simulink model "lane_departure"  (R2017a)
settings: Solver=FixedStepDiscrete  StartTime=0.0  StopTime=inf  FixedStep=1/50  RelTol=1e-3  EnableMultiTasking=on
libraries: visionsinks x1, dspvision x1, embdlinuxlib x1
settings Model: Creator=ChiChaChai  LastModifiedBy=ChiChaChai
settings SolverCC: PositivePriorityOrder=on  AutoInsertRateTranBlk=on
settings OptimizationCC: UseFloatMulNetSlope=on  PassReuseOutputArgsAs=Individual arguments  ZeroExternalMemoryAtStartup=off  ZeroInternalMemoryAtStartup=off  NoFixptDivByZeroProtection=on  EfficientFloat2IntCast=on  LifeSpan=1  MaxStackSize=64
settings DebuggingCC: ParameterTunabilityLossMsg=error
settings HardwareCC: ProdBitPerPointer=32  ProdBitPerSizeT=32  ProdBitPerPtrDiffT=32  ProdLargestAtomicInteger=Long  ProdLargestAtomicFloat=Double  ProdWordSize=32  ProdHWDeviceType=ARM Compatible->ARM Cortex
settings ModelReferenceCC: PropagateVarSize=Only when enabling
settings SFSimCC: MATLABDynamicMemAlloc=off
settings RTWCC: SystemTargetFile=ert.tlc  HardwareBoard=Raspberry Pi  TLCOptions="-aInlineSetEventsForThisBaseRateFcn=TLC_FALSE -aSuppressMultiTaskScheduler=TLC_FALSE  -aRateBasedStepFcn=0"  TemplateMakefile=ert_default_tmf  Description=Embedded Coder  GenerateReport=on  Toolchain=GNU GCC Raspberry Pi  IncludeHyperlinkInReport=on  LaunchReport=on  GenerateTraceInfo=on  GenerateTraceReport=on  GenerateTraceReportSl=on  GenerateTraceReportSf=on  GenerateTraceReportEml=on  GenerateCodeMetricsReport=on
settings CodeAppCC: ForceParamTrailComments=on  IgnoreCustomStorageClasses=off  OperatorAnnotations=on  SimulinkDataObjDesc=on  SFDataObjDesc=on  MATLABFcnDesc=on  CustomSymbolStrGlobalVar=rt$N$M  CustomSymbolStrType=$N$M  CustomSymbolStrFcn=$N$M$F  CustomSymbolStrMacro=$N$M  InsertBlockDesc=on  MATLABSourceComments=on
settings ERTTargetCC: IncludeMdlTerminateFcn=off  CombineSignalStateStructs=on  SupportAbsoluteTime=off  SupportComplex=off  SupportNonInlinedSFcns=on  SupportVariableSizeSignals=on  ExtMode=on  ExtModeMexArgs='192.168.1.228' 0 17725  ERTFilePackagingFormat=CompactWithDataFile

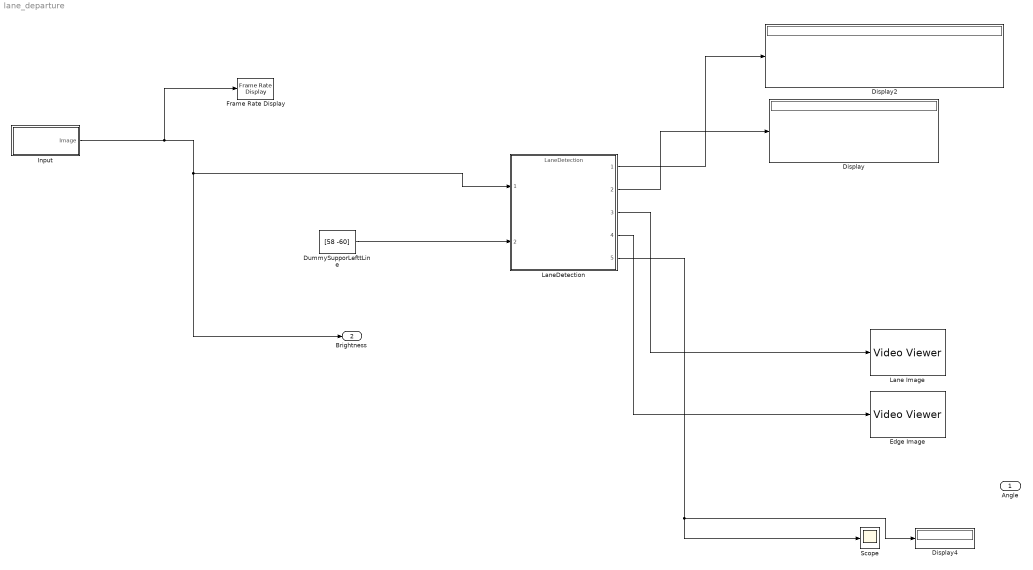
== system lane_departure ==
  Display : Display
  Display2 : Display
  Display4 : Display
  DummySupporLefttLine : Constant  Value=[58 -60]  VectorParams1D=off  OutDataTypeStr=double
  Edge Image : VideoViewer  FigPos=[1033.8 504.4 304 248]
  Frame Rate Display : visionsinks/Frame Rate Display  UpdateRate=10
      settings: SourceProductName=Computer Vision System Toolbox  SourceProductBaseCode=VP
  "Input " : Subsystem
  Lane Image : VideoViewer  FigPos=[301.8 784.4 343.2 246.4]
  LaneDetection : ModelReference  ModelNameDialog=LaneDetection  SimulationMode=Normal  ModelReferenceVersion=1.287
  Scope : Scope
  Angle : Outport
  Brightness : Outport  Port=2
  wires:
  LaneDetection/3 -> Lane Image/1
  LaneDetection/4 -> Edge Image/1
  LaneDetection/2 -> Display/1
  DummySupporLefttLine/1 -> LaneDetection/2
  LaneDetection/5 -> Scope/1, Display4/1
  LaneDetection/1 -> Display2/1
  "Input "/1(Image) -> Brightness/1, LaneDetection/1, Frame Rate Display/1

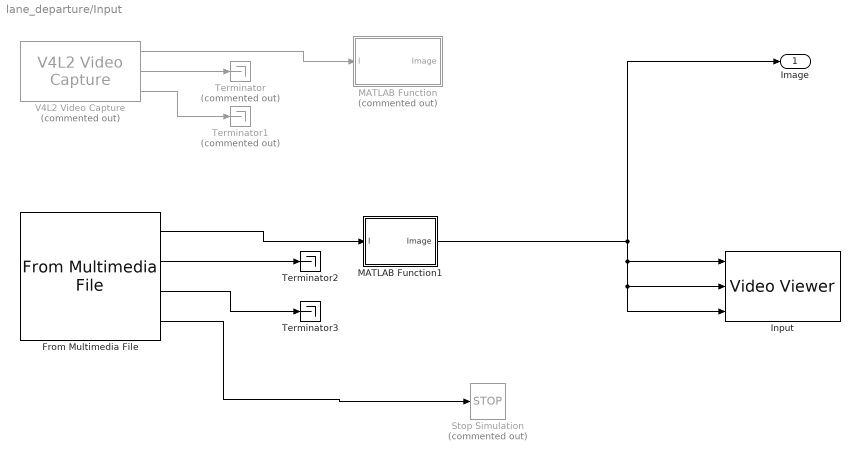
== system lane_departure/Input  ==
  From Multimedia File : dspvision/From Multimedia File  inputFilename=C:\Users\ChiChaChai\Documents\AMAS-2017\SelfDrivingCar_with_MATLAB\testing_src\video6.mp4  loop=on  numPlays=inf  outputStreams=Video only  videoDataType=uint8  audioDataType=int16  inheritSampleTime=off  userDefinedSampleTime=1/25  noAudioOutput=off  isIntensityVideo=off  fourcc=YCbCr 4:2:2  colorVideoFormat=One multidimensional signal  outputEOF=on  dataOrg=Column-major  audioFrameSize=1024  computeAudioFrameSize=off  outSamplingMode=Sample based
      settings: SourceProductBaseCode=VP
  Input : VideoViewer  imagePorts=separate color signals  FigPos=[1.8 450 317.6 247.2]
  MATLAB Function : MATLAB Function  Commented=on  TreatAsAtomicUnit=on
  MATLAB Function1 : MATLAB Function  TreatAsAtomicUnit=on
  Stop Simulation : Stop  Commented=on
  Terminator : Terminator  Commented=on
  Terminator1 : Terminator  Commented=on
  Terminator2 : Terminator
  Terminator3 : Terminator
  V4L2 Video Capture : embdlinuxlib/V4L2 Video Capture  Commented=on  m_devName='/dev/video0'  roi=[0, 0, 640, 480]  imSizeSelection=320x240  imSize=[640, 480]  pixelFormat=YCbCr 4:2:2  pixelOrder=Planar  sampleTime=1/50  simOutput=Colorbars  blockPlatform=Raspberry Pi
  Image : Outport
  wires:
  V4L2 Video Capture/2 -> Terminator/1
  V4L2 Video Capture/3 -> Terminator1/1
  V4L2 Video Capture/1 -> MATLAB Function/1(I)
  From Multimedia File/2 -> Terminator2/1
  From Multimedia File/3 -> Terminator3/1
  From Multimedia File/1 -> MATLAB Function1/1(I)
  From Multimedia File/4 -> Stop Simulation/1
  MATLAB Function1/1(Image) -> Input/3, Input/2, Input/1, Image/1

== matlab function lane_departure/Input /MATLAB Function1 ==
  data: I input; Image output
function Image = Flip(I)

Image = imrotate(I,180,'bilinear');

== matlab function lane_departure/Input /MATLAB Function ==
  data: I input; Image output
function Image = FlipAndRotate(I)
Image = imrotate(I,90,'bilinear');
Image = flip(Image,2);
